simulink model "sensorExpoler_hall_sensor"  (R2026a)
settings: Solver=FixedStepAuto  StopTime=5  FixedStep=0.001
undefined symbols (not defined in the file or in its folder): Blocking, Non
libraries: amg_usbconverter_n_connect_lib x2
settings Model: Creator=pboon  LastModifiedBy=acer

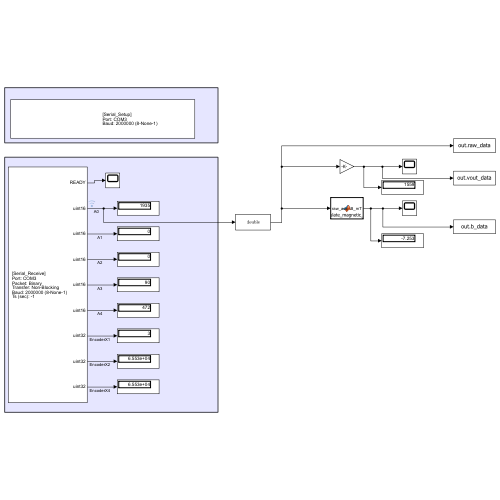
[thumbnail: Simulink's stored preview of the top-level diagram]
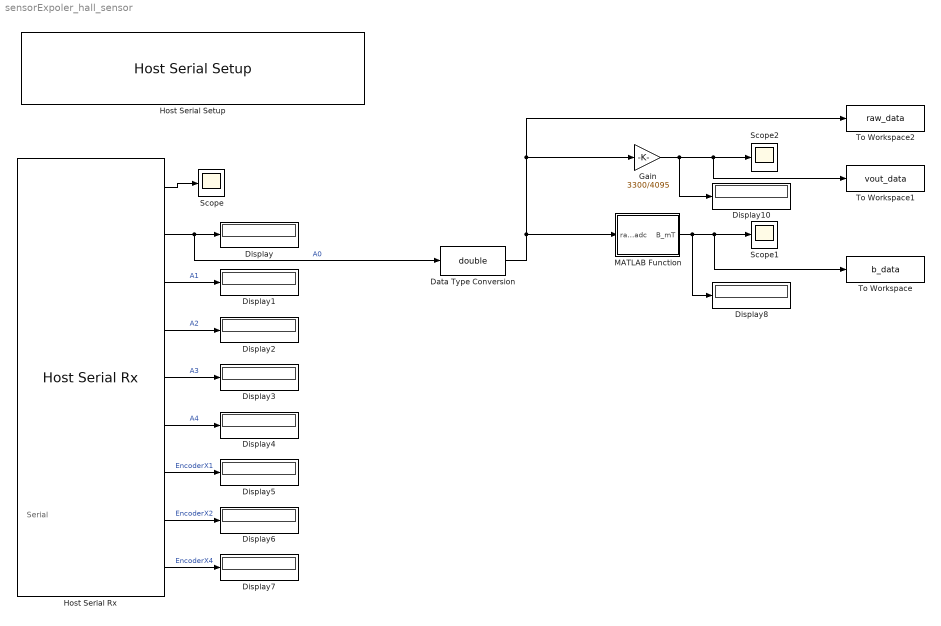
== system sensorExpoler_hall_sensor ==
  note: Serial
  Data Type Conversion : DataTypeConversion  OutDataTypeStr=double  SaturateOnIntegerOverflow=off  RndMeth=Floor  LockScale=on
  Display{,1..8,10} (10 alike) : Display
  Gain : Gain  Gain=3300/4095
  Host Serial Rx : amg_usbconverter_n_connect_lib/Host Serial Rx  conf=rx  port=<auto>  baudrate=2000000  databits=8  parity=None  stopbit=1  flowcontrol=None  transfer=Non-Blocking  timeout=5  packetmode=Binary  enableinitialvalues=off  initialvalues=[]  binheader='25'  binterminator='4E 4E'  porttype_double=0  porttype_single=0  porttype_int8=0  porttype_uint8=0  porttype_int16=0  porttype_uint16=5  porttype_int32=0  porttype_uint32=3  asciiformat='%d,%f'  rx_asciiterminator="CRLF (0x0D 0x0A - \"\\r\\n\")"  tx_asciiterminator="CRLF (0x0D 0x0A - \"\\r\\n\")"  sampletime=0.001  enablecustomportlabel=off  cinputportlabel=0  coutputportlabel=A  portpinstr=0  blockid=HostSerialRx  inputporttype=[]  inputportwidth=[]  inputportlabel={}  outputporttype=[3 5 5 5 5 5 7 7 7]  outputportwidth=[1 1 1 1 1 1 1 1 1]  outputportlabel={'READY','uint16','uint16','uint16','uint16','uint16','uint32','uint32','uint32'}  compat=0  optionstring=[]  autoport='COM3'
  Host Serial Setup : amg_usbconverter_n_connect_lib/Host Serial Setup  conf=setup  port=<auto>  baudrate=2000000  databits=8  parity=None  stopbit=1  flowcontrol=None  transfer=Blocking  timeout=2  packetmode=Binary  initialvalues=[]  binheader='7E 7E'  binterminator='03 03'  porttype_double=0  porttype_single=1  porttype_int8=0  porttype_uint8=0  porttype_int16=0  porttype_uint16=0  porttype_int32=0  porttype_uint32=2  asciiformat='%d %u %x'  rx_asciiterminator="CRLF (0x0D 0x0A - \"\\r\\n\")"  tx_asciiterminator="CRLF (0x0D 0x0A - \"\\r\\n\")"  sampletime=-1  enablecustomportlabel=off  cinputportlabel=0  coutputportlabel=A  portpinstr=0  blockid=HostSerialSetup  inputporttype=[]  inputportwidth=[]  inputportlabel={}  outputporttype=[]  outputportwidth=[]  outputportlabel={}  compat=0  optionstring=[]  autoport='COM3'
  MATLAB Function : MATLAB Function  TreatAsAtomicUnit=on
  Scope : Scope
      settings: ActiveDisplayYMinimum=-0.12499999999999997  ActiveDisplayYMaximum=1.125
  Scope1 : Scope
      settings: ActiveDisplayYMinimum=-49.254212454212464  ActiveDisplayYMaximum=-47.642490842490844
  Scope2 : Scope
      settings: ActiveDisplayYMinimum=927.245454788208  ActiveDisplayYMaximum=1123.6744213104248  DataLoggingVariableName=ScopeData2
  To Workspace : ToWorkspace  VariableName=b_data  SampleTime=-1
  To Workspace1 : ToWorkspace  VariableName=vout_data  SampleTime=-1
  To Workspace2 : ToWorkspace  VariableName=raw_data  SampleTime=-1
  wires:
  Host Serial Rx/2 -> Data Type Conversion/1, Display/1  "A0"
  Host Serial Rx/3 -> Display1/1  "A1"
  Host Serial Rx/4 -> Display2/1  "A2"
  Host Serial Rx/5 -> Display3/1  "A3"
  Host Serial Rx/6 -> Display4/1  "A4"
  Host Serial Rx/7 -> Display5/1  "EncoderX1"
  Host Serial Rx/8 -> Display6/1  "EncoderX2"
  Host Serial Rx/9 -> Display7/1  "EncoderX4"
  Host Serial Rx/1 -> Scope/1
  MATLAB Function/1(B_mT) -> Display8/1, To Workspace/1, Scope1/1
  Gain/1 -> Display10/1, To Workspace1/1, Scope2/1
  Data Type Conversion/1 -> To Workspace2/1, Gain/1, MATLAB Function/1(raw_adc)

== matlab function sensorExpoler_hall_sensor/MATLAB Function ==
  data: raw_adc input; B_mT output
function B_mT = calculate_magnetic_flux(raw_adc)
    % 1. กำหนดค่าคงที่ของระบบ (System Constants)
    V_ref = 3300;       % แรงดันไฟเลี้ยงอ้างอิงของบอร์ด STM32 (mV)
    ADC_res = 4095;     % ความละเอียด ADC 12-bit (0-4095)
    
    % 2. กำหนดค่าคงที่จาก Datasheet ของ DRV5055 (ต้องเปลี่ยนค่าให้ตรงกับรุ่นที่ใช้)
    V_Q = 1650;         % แรงดันไฟฟ้าขาออกขณะไม่มีสนามแม่เหล็ก (mV)
    Sens_25 = 12.5;     % ค่า Sensitivity ที่ 25 องศาเซลเซียส (mV/mT) -> เช็กจากรุ่น A1-A4
    S_TC = 0.12 / 100;  % ค่าสัมประสิทธิ์อุณหภูมิ 
    T_A = 25;           % อุณหภูมิแวดล้อมขณะทดลอง (องศาเซลเซียส)

    % 3. แปลงค่า Raw ADC เป็นแรงดันไฟฟ้า V_out (mV)
    V_out = (raw_adc / ADC_res) * V_ref;

    % 4. คำนวณความเข้มสนามแม่เหล็ก B (mT) ตามสมการ
    % V_out = V_Q + B * (Sens_25 * (1 + S_TC * (T_A - 25)))
    
    denominator = Sens_25 * (1 + (S_TC * (T_A - 25)));
    
    % ป้องกัน Error กรณีตัวหารเป็น 0
    if denominator == 0
        B_mT = 0;
    else
        B_mT = (V_out - V_Q) / denominator;
    end
end
